simulink model "joint_1_PID_controller"  (R2025a)
settings: Solver=VariableStepAuto  StartTime=0.0  StopTime=10.0  RelTol=1e-3
undefined symbols (not defined in the file or in its folder): Kd1, Ki1, Kp1
settings Model: Creator=nethi  LastModifiedBy=nethi

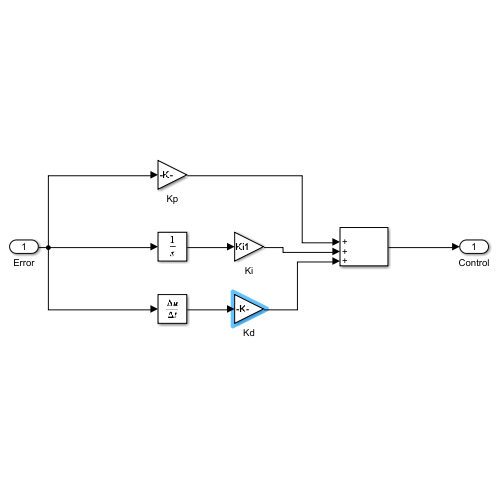
[thumbnail: Simulink's stored preview of the top-level diagram]
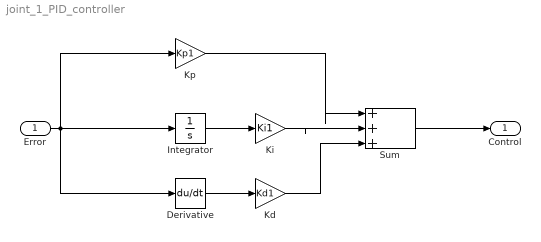
== system joint_1_PID_controller ==
  Error : Inport
  Derivative : Derivative
  Integrator : Integrator
  Kd : Gain  Gain=Kd1
  Ki : Gain  Gain=Ki1
  Kp : Gain  Gain=Kp1
  Sum : Sum  Inputs=|+++
  Control : Outport
  wires:
  Error/1 -> Derivative/1, Kp/1, Integrator/1
  Integrator/1 -> Ki/1
  Derivative/1 -> Kd/1
  Ki/1 -> Sum/2
  Kp/1 -> Sum/1
  Sum/1 -> Control/1
  Kd/1 -> Sum/3
